simulink model "red_dim_observer"  (R2020b)
settings: Solver=VariableStepAuto  StartTime=0.0  StopTime=10.0  RelTol=1e-3
settings Model: Creator=10853  LastModifiedBy=10853

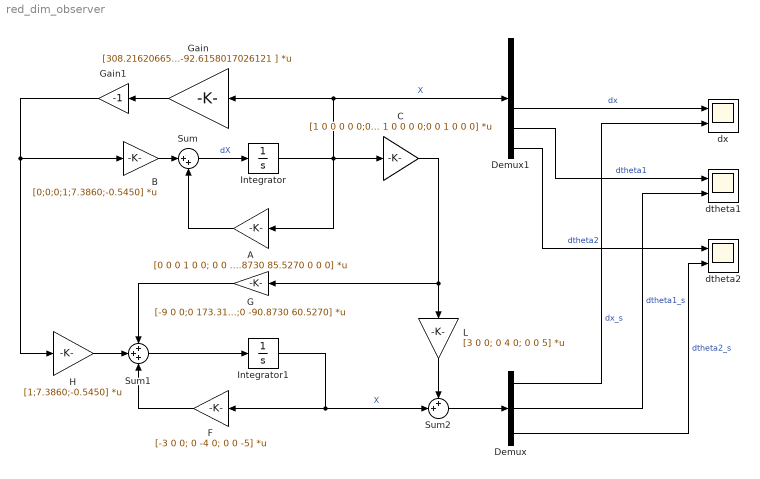
== system red_dim_observer ==
  A : Gain  Gain=[0 0 0 1 0 0; 0 0 0 0 1 0; 0 0 0 0 0 1;0 0 0 0 0 0; 0 189.318 -116.9320 0 0 0; 0 -90.8730 85.5270 0 0 0]  Multiplication=Matrix(K*u)
  B : Gain  Gain=[0;0;0;1;7.3860;-0.5450]  Multiplication=Matrix(K*u)
  C : Gain  Gain=[1 0 0 0 0 0;0 1 0 0 0 0;0 0 1 0 0 0]  Multiplication=Matrix(K*u)
  Demux : Demux  Outputs=3
  Demux1 : Demux  Outputs=6
  F : Gain  Gain=[-3 0 0; 0 -4 0; 0 0 -5]  Multiplication=Matrix(K*u)
  G : Gain  Gain=[-9 0 0;0 173.3180 -116.9320;0 -90.8730 60.5270]  Multiplication=Matrix(K*u)
  Gain : Gain  Gain=|  Multiplication=Matrix(K*u)
      | [308.216206651111	158.619423985671	-617.386289524257	151.829835967496	-19.2479620762821	-92.6158017026121
      | ]
  Gain1 : Gain  Gain=-1
  H : Gain  Gain=[1;7.3860;-0.5450]  Multiplication=Matrix(K*u)
  Integrator : Integrator  InitialCondition=[0;pi/36;pi/36;0;0;0]
  Integrator1 : Integrator  InitialCondition=[0;0;0]
  L : Gain  Gain=[3 0 0; 0 4 0; 0 0 5]  Multiplication=Matrix(K*u)
  Sum : Sum  Inputs=|++
  Sum1 : Sum  Inputs=+++
  Sum2 : Sum  Inputs=++|
  dtheta1 : Scope  NumInputPorts=2
  dtheta2 : Scope  NumInputPorts=2
  dx : Scope  NumInputPorts=2
  wires:
  Sum/1 -> Integrator/1  "dX"
  B/1 -> Sum/1
  Integrator/1 -> Gain/1, Demux1/1, A/1, C/1  "X"
  A/1 -> Sum/2
  C/1 -> L/1, G/1
  G/1 -> Sum1/1
  H/1 -> Sum1/2
  Sum1/1 -> Integrator1/1
  F/1 -> Sum1/3
  Integrator1/1 -> Sum2/2, F/1  "X"
  L/1 -> Sum2/1
  Gain/1 -> Gain1/1
  Gain1/1 -> H/1, B/1
  Sum2/1 -> Demux/1
  Demux/1 -> dx/2  "dx_s"
  Demux1/5 -> dtheta1/1  "dtheta1"
  Demux/2 -> dtheta1/2  "dtheta1_s"
  Demux1/6 -> dtheta2/1  "dtheta2"
  Demux/3 -> dtheta2/2  "dtheta2_s"
  Demux1/4 -> dx/1  "dx"
